simulink model "BuckConverter_iDesignMask"  (R2020b)
settings: Solver=FixedStepAuto  StartTime=0.0  StopTime=100  FixedStep=0.0015  RelTol=1e-3
libraries: PB_Library_Master x1, Lib_Solve_SSNRSolverJC_EMTAT x1
settings Model: Creator=pmatt  LastModifiedBy=nbutler2
settings SFSimCC: CustomCodeUndefinedFunction=UseInterfaceOnly

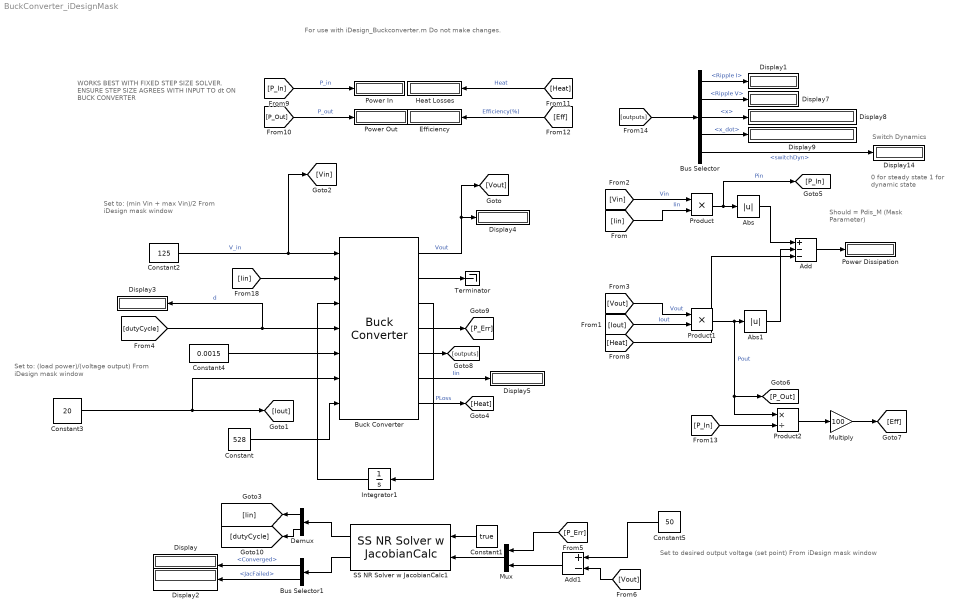
== system BuckConverter_iDesignMask ==
  note: WORKS BEST WITH FIXED
      | STEP SIZE SOLVER. ENSURE
      | STEP SIZE AGREES WITH INPUT
      | TO dt ON BUCK CONVERTER
  note: Set to:
      | (load power)/(voltage output)
      | From iDesign mask window
  note: Set to desired output voltage (set point)
      | From iDesign mask window
  note: Switch Dynamics
  note: Should = Pdis_M
      | (Mask Parameter)
  note: For use with iDesign_Buckconverter.m
      | Do not make changes.
  note: 0 for steady state
      | 1 for dynamic state
  note: Set to:
      | (min Vin + max Vin)/2
      | From iDesign mask window
  Abs : Abs
  Abs1 : Abs
  Add : Sum  Inputs=+--
  Add1 : Sum  Inputs=+-
  Buck Converter : PB_Library_Master/Buck Converter  Pdis_M=1  C_M=4.07e-07  L_M=6e-05  Ron_M=0.0009  RC_M=0.030919  RL_M=0.019013  QgTotal_M=5.8e-08  Vgate_M=1.9  TRise_M=2.2e-08  TFall_M=4.4e-08  Fsw_M=250000  Trr_M=7.7e-08  n_MOSFET=1  MassEst_M=3.7515  TempIn=Celsius  vOut=50  pow=1000  minV=123  maxV=127  rippleMode=Use defaults (5% of voltage output and 10% of inductor current)  vRip=.05  iRip=.1  freqMode=Use default frequency (250 kHz)  freq=250e3
  Bus Selector : BusSelector  OutputSignals=Ripple I,Ripple V,x,x_dot,switchDyn
  Bus Selector1 : BusSelector  OutputSignals=Converged,JacFailed
  Constant : Constant  Value=528
  Constant1 : Constant  Value=true
  Constant2 : Constant  Value=125  VectorParams1D=off  SampleTime=-1
  Constant3 : Constant  Value=20
  Constant4 : Constant  Value=0.0015  VectorParams1D=off
  Constant5 : Constant  Value=50
  Demux : Demux  Outputs=2
  Display{,1..5,7..9,14} (10 alike) : Display
      Display8 settings: Decimation=3
  Efficiency : Display
  Heat Losses : Display
  Integrator1 : Integrator  InitialCondition=[0;0]
  Multiply : Gain  Gain=100
  Mux : Mux  Inputs=2
  Power Dissipation : Display
  Power In : Display
  Power Out : Display
  Product : Product
  Product1 : Product
  Product2 : Product  Inputs=*/
  SS NR Solver w JacobianCalc1 : Lib_Solve_SSNRSolverJC_EMTAT/SS NR Solver w JacobianCalc  SJac_Per_M=[.01, .001; -.01, -.001]  SNR_IC_M=[5;0.5]  SNR_DX_M=[100000;0.99999]  SNR_Mx_M=100000  SNR_Mn_M=[0.00001;0.00001]  SJacobianAttempts_M=200  Cond_Limits_M=0.0001
  Terminator : Terminator
  wires:
  [Iin] -> Buck Converter/2
  [Eff] -> Efficiency/1  "Efficiency(%)"
  Integrator1/1 -> Buck Converter/3
  Buck Converter/4 -> [P_Err]
  Buck Converter/5 -> [outputs]
  [Vout] -> Product1/1  "Vout"
  Constant2/1 -> Buck Converter/1, [Vin]  "V_in"
  Bus Selector/2 -> Display7/1  "<Ripple V>"
  Bus Selector/5 -> Display14/1  "<switchDyn>"
  Bus Selector/4 -> Display9/1  "<x_dot>"
  Buck Converter/7 -> [Heat]  "PLoss"
  [Iin] -> Product/2  "Iin"
  Buck Converter/6 -> Display5/1  "Iin"
  [Iout] -> Product1/2  "Iout"
  [P_Out] -> Power Out/1  "P_out"
  Abs1/1 -> Add/2
  Abs/1 -> Add/1
  [outputs] -> Bus Selector/1
  Bus Selector/1 -> Display1/1  "<Ripple I>"
  Buck Converter/3 -> Integrator1/1
  [Vin] -> Product/1  "Vin"
  [Heat] -> Heat Losses/1  "Heat"
  Bus Selector/3 -> Display8/1  "<x>"
  [P_In] -> Product2/2
  Add/1 -> Power Dissipation/1
  Product/1 -> [P_In], Abs/1  "Pin"
  Buck Converter/1 -> [Vout], Display4/1  "Vout"
  Multiply/1 -> [Eff]
  Product2/1 -> Multiply/1
  [P_In] -> Power In/1  "P_in"
  Product1/1 -> [P_Out], Product2/1, Abs1/1  "Pout"
  Constant/1 -> Buck Converter/7
  Buck Converter/2 -> Terminator/1
  Constant3/1 -> Buck Converter/6, [Iout]
  [Heat] -> Add/3
  Constant4/1 -> Buck Converter/5
  [dutyCycle] -> Buck Converter/4, Display3/1  "d"
  Constant1/1 -> SS NR Solver w JacobianCalc1/1
  SS NR Solver w JacobianCalc1/2 -> Bus Selector1/1
  Bus Selector1/1 -> Display/1  "<Converged>"
  Bus Selector1/2 -> Display2/1  "<JacFailed>"
  SS NR Solver w JacobianCalc1/1 -> Demux/1
  Demux/1 -> [Iin]
  Demux/2 -> [dutyCycle]
  [Vout] -> Add1/2
  Constant5/1 -> Add1/1
  Add1/1 -> Mux/2
  [P_Err] -> Mux/1
  Mux/1 -> SS NR Solver w JacobianCalc1/2
